simulink model "StateController"  (R2024a)
settings: Solver=VariableStepAuto  StartTime=0.0  StopTime=10.0  RelTol=1e-3
settings Model: DataDictionary=SysMLArchModel_DD.sldd  Creator=ykamatan  LastModifiedBy=ykamatan

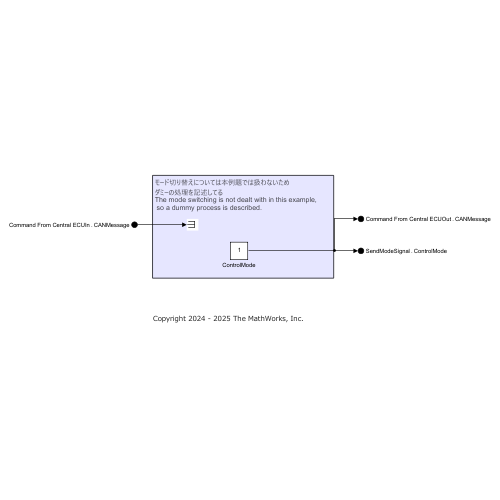
[thumbnail: Simulink's stored preview of the top-level diagram]
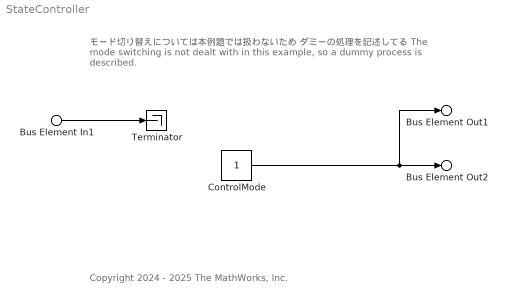
== system StateController ==
  note: モード切り替えについては本例題では扱わないため
      | ダミーの処理を記述してる
      | The mode switching is not dealt with in this example,
      |  so a dummy process is described.
  note: Copyright 2024 - 2025 The MathWorks, Inc.
  Bus Element In1 : Inport  PortName=Command From Central ECUIn  Element=CANMessage
  ControlMode : Constant
  Terminator : Terminator
  Bus Element Out1 : Outport  PortName=Command From Central ECUOut  Element=CANMessage
  Bus Element Out2 : Outport  Port=2  PortName=SendModeSignal  Element=ControlMode
  wires:
  Bus Element In1/1 -> Terminator/1
  ControlMode/1 -> Bus Element Out2/1, Bus Element Out1/1
